simulink model "caso_non_noto_con_ingresso"  (R2024b)
settings: Solver=VariableStepAuto  StartTime=0.0  StopTime=25.0  MaxStep=1e-4  RelTol=1e-5
settings Model: Creator=david  LastModifiedBy=david

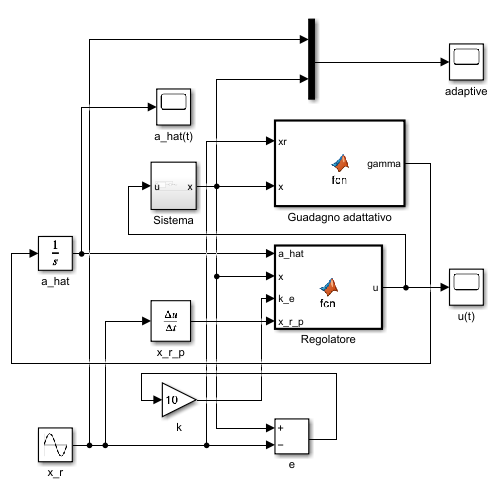
[thumbnail: Simulink's stored preview of the top-level diagram]
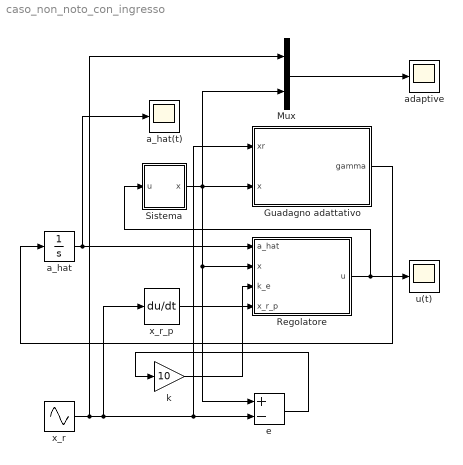
== system caso_non_noto_con_ingresso ==
  Guadagno adattativo : MATLAB Function  TreatAsAtomicUnit=on
  Mux : Mux  Inputs=2
  Regolatore : MATLAB Function  TreatAsAtomicUnit=on
  Sistema : Subsystem
  a_hat : Integrator
  a_hat(t) : Scope
  adaptive : Scope
  e : Sum  Inputs=+-
  k : Gain  Gain=10
  u(t) : Scope
  x_r : Sin  SampleTime=0
  x_r_p : Derivative
  wires:
  x_r_p/1 -> Regolatore/4(x_r_p)
  a_hat/1 -> a_hat(t)/1, Regolatore/1(a_hat)
  Guadagno adattativo/1(gamma) -> a_hat/1
  x_r/1 -> e/2, Guadagno adattativo/1(xr), x_r_p/1, Mux/1
  Sistema/1(x) -> e/1, Regolatore/2(x), Mux/2, Guadagno adattativo/2(x)
  k/1 -> Regolatore/3(k_e)
  Mux/1 -> adaptive/1
  Regolatore/1(u) -> u(t)/1, Sistema/1(u)
  e/1 -> k/1

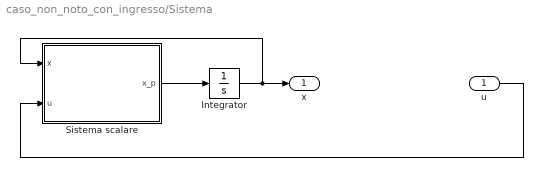
== system caso_non_noto_con_ingresso/Sistema ==
  u : Inport
  Integrator : Integrator
  Sistema scalare : MATLAB Function  TreatAsAtomicUnit=on
  x : Outport
  wires:
  u/1 -> Sistema scalare/2(u)
  Integrator/1 -> Sistema scalare/1(x), x/1
  Sistema scalare/1(x_p) -> Integrator/1

== matlab function caso_non_noto_con_ingresso/Regolatore ==
  data: a_hat input; x input; u output; k_e input; x_r_p input
function u = fcn(a_hat,x,k_e,x_r_p)



u = -a_hat*x + x_r_p - k_e;%regolazione

== matlab function caso_non_noto_con_ingresso/Sistema/Sistema scalare ==
  data: x input; x_p output; u input
function x_p = fcn(x,u)

a=10;
x_p = a*x+u;

== matlab function caso_non_noto_con_ingresso/Guadagno adattativo ==
  data: xr input; x input; gamma output
function gamma = fcn(xr,x)

gamma = 10*((x-xr)*x);
